simulink model "Gantry1DSimulink_V4"  (R2024b)
settings: Solver=FixedStepAuto  StartTime=0.0  StopTime=inf  FixedStep=0.05  RelTol=1e-3  EnableMultiTasking=on
undefined symbols (not defined in the file): DiscIntNeverNeededParam
libraries: raspberrypiBasiclib x5, raspberrypiNetworklib x5, etargetslib x1, simulink x1
settings Model: ExtModeTrigDuration=2  Creator=ioannisgeorgilas  LastModifiedBy=oskarchu
settings SolverCC: PositivePriorityOrder=on
settings OptimizationCC: EnhancedBackFolding=on  PassReuseOutputArgsAs=Individual arguments  ZeroExternalMemoryAtStartup=off  ZeroInternalMemoryAtStartup=off  MaxStackSize=200000  OptimizeBlockOrder=speed  DifferentSizesBufferReuse=on  OptimizationCustomize=off  EfficientTunableParamExpr=on
settings DebuggingCC: ParameterTunabilityLossMsg=error
settings HardwareCC: ProdBitPerPointer=32  ProdBitPerSizeT=32  ProdBitPerPtrDiffT=32  ProdLargestAtomicInteger=Long  ProdLargestAtomicFloat=Double  ProdWordSize=32  ProdLongLongMode=on  ProdHWDeviceType=ARM Compatible->ARM Cortex-A (32-bit)
settings RTWCC: Description=Embedded Coder  SystemTargetFile=ert.tlc  HardwareBoard=Raspberry Pi  TLCOptions="-aInlineSetEventsForThisBaseRateFcn=TLC_FALSE -aSuppressMultiTaskScheduler=TLC_FALSE  -aRateBasedStepFcn=0"  TemplateMakefile=ert_default_tmf  Toolchain=GNU GCC Embedded Linux  BuildConfiguration=Faster Runs
settings CodeAppCC: ForceParamTrailComments=on  IgnoreCustomStorageClasses=off  OperatorAnnotations=on  SimulinkDataObjDesc=on  SFDataObjDesc=on  InsertBlockDesc=on
settings ERTTargetCC: CodeReplacementLibrary=ARM Cortex-A CMSIS  SupportVariableSizeSignals=on  ExtModeTransport=2  ExtModeStaticAlloc=on  ExtModeMexFile=ext_xcp  ExtModeIntrfLevel=Level2 - Open  InlinedParameterPlacement=Hierarchical

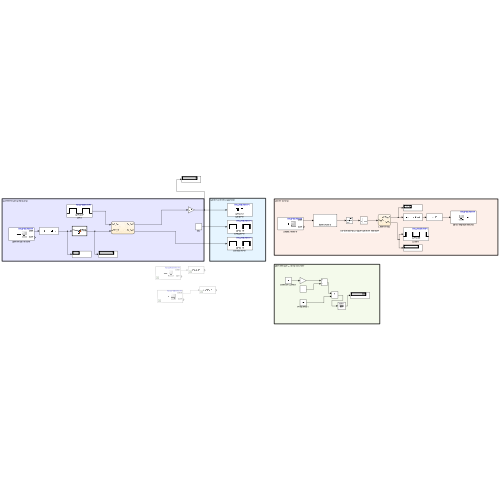
[thumbnail: Simulink's stored preview of the top-level diagram]
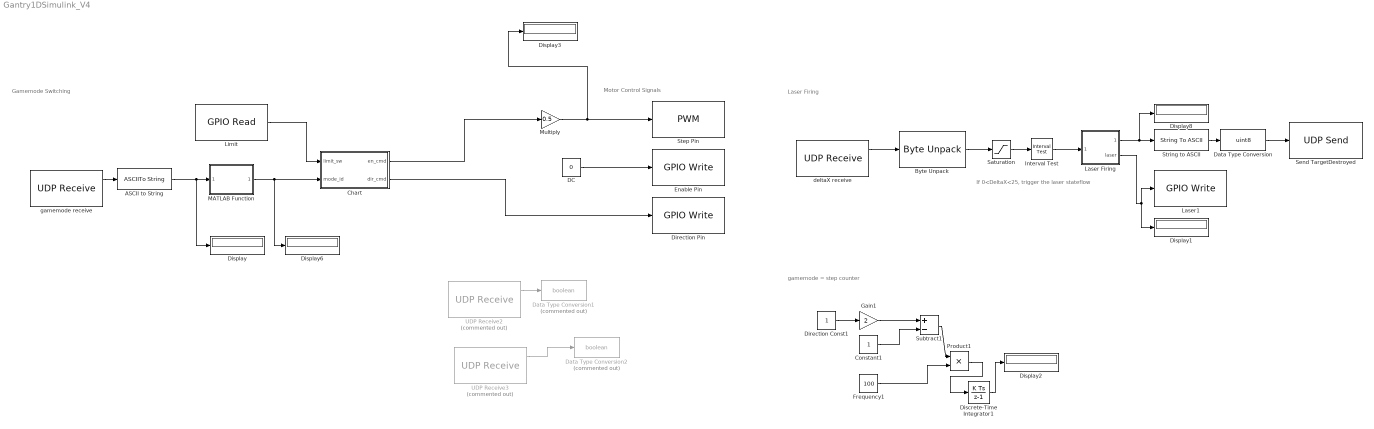
== system Gantry1DSimulink_V4 ==
  note: If 0<DeltaX<25, trigger the laser stateflow
  note: Motor Control Signals
  note: gamemode = step counter
  note: Laser Firing
  note: Gamemode Switching
  ASCII to String : ASCIIToString
  Byte Unpack : etargetslib/Byte Unpack  dimensions={[1]}  datatypes={'int32'}  byteAlign=1
      settings: LibrarySourceBlock=embeddedtargetslib/Host Communication/Byte Unpack
  Chart : Stateflow chart  TreatAsAtomicUnit=on
  Constant1 : Constant
  DC : Constant  Value=0
  Data Type Conversion : DataTypeConversion  OutDataTypeStr=uint8  SaturateOnIntegerOverflow=off  RndMeth=Floor
  Data Type Conversion1 : DataTypeConversion  Commented=on  OutDataTypeStr=boolean  SaturateOnIntegerOverflow=off  RndMeth=Floor
  Data Type Conversion2 : DataTypeConversion  Commented=on  OutDataTypeStr=boolean  SaturateOnIntegerOverflow=off  RndMeth=Floor
  Direction Const1 : Constant
  Direction Pin : raspberrypiBasiclib/GPIO Write  BoardProperty=Pi Zero 2 W  gpio=14  blockPlatform=Raspberry Pi  PinNumber=17  board=[]  direction=[]
  Discrete-Time Integrator1 : DiscreteIntegrator  SampleTime=-1  ICPrevOutput=DiscIntNeverNeededParam  ICPrevScaledInput=DiscIntNeverNeededParam
  Display{,1..3,6,8} (6 alike) : Display
  Enable Pin : raspberrypiBasiclib/GPIO Write  BoardProperty=Pi Zero 2 W  gpio=19  blockPlatform=Raspberry Pi  PinNumber=17  board=[]  direction=[]
  Frequency1 : Constant  Value=100
  Gain1 : Gain  Gain=2
  Interval Test : simulink/Logic and Bit Operations/Interval Test  IntervalClosedRight=on  uplimit=25  IntervalClosedLeft=on  lowlimit=0  OutDataTypeStr=boolean
  Laser Firing : Stateflow chart  TreatAsAtomicUnit=on
  Laser1 : raspberrypiBasiclib/GPIO Write  BoardProperty=Pi Zero 2 W  gpio=22  blockPlatform=Raspberry Pi  PinNumber=17  board=[]  direction=[]
  Limit : raspberrypiBasiclib/GPIO Read  BoardProperty=Pi Zero 2 W  gpio=27  SampleTime=0.05  blockPlatform=Raspberry Pi  PinNumber=4  board=[]  direction=[]  internalResistor=[]
  MATLAB Function : MATLAB Function  TreatAsAtomicUnit=on
  Multiply : Gain  Gain=0.5
  Product1 : Product
  Saturation : Saturate  UpperLimit=500  LowerLimit=-500
  Send TargetDestroyed : raspberrypiNetworklib/UDP Send  remoteURL='172.26.236.65'  remotePort=55004  localURL='0.0.0.0'  localPortSource=Automatically determine  localPort=-1  sampletime=-1  blockPlatform=Raspberry Pi  separateLengthPort=0
      settings: SourceProductName=Network
  Step Pin : raspberrypiBasiclib/PWM  board=Pi Zero W  Pin_=12  Frequency=200  blockPlatform=Raspberry Pi
  String to ASCII : StringToASCII
  Subtract1 : Sum  Inputs=+-
  UDP Receive2 : raspberrypiNetworklib/UDP Receive  Commented=on  localURL='0.0.0.0'  localPort=50001  remoteURL='0.0.0.0'  remotePort=-1  recvBufferSize=8192  signalDatatype=uint8  dims=1  isVarSize=off  showBlockingTime=off  blockingTime=0  sampletime=1  blockPlatform=Raspberry Pi
      settings: SourceProductName=Network
  UDP Receive3 : raspberrypiNetworklib/UDP Receive  Commented=on  localURL='0.0.0.0'  localPort=50002  remoteURL='0.0.0.0'  remotePort=-1  recvBufferSize=8192  signalDatatype=uint8  dims=1  isVarSize=off  showBlockingTime=off  blockingTime=0  sampletime=1  blockPlatform=Raspberry Pi
      settings: SourceProductName=Network
  deltaX receive : raspberrypiNetworklib/UDP Receive  localURL='0.0.0.0'  localPort=55010  remoteURL='0.0.0.0'  remotePort=-1  recvBufferSize=8192  signalDatatype=uint8  dims=4  isVarSize=off  showBlockingTime=off  blockingTime=0  sampletime=0.05  blockPlatform=Raspberry Pi
      settings: SourceProductName=Network
  gamemode receive : raspberrypiNetworklib/UDP Receive  localURL='0.0.0.0'  localPort=50001  remoteURL='0.0.0.0'  remotePort=-1  recvBufferSize=8192  signalDatatype=uint8  dims=14  isVarSize=off  showBlockingTime=off  blockingTime=0  sampletime=0.05  blockPlatform=Raspberry Pi
      settings: SourceProductName=Network
  wires:
  UDP Receive3/1 -> Data Type Conversion2/1
  UDP Receive2/1 -> Data Type Conversion1/1
  Chart/2(dir_cmd) -> Direction Pin/1
  Discrete-Time Integrator1/1 -> Display2/1
  Product1/1 -> Discrete-Time Integrator1/1
  Direction Const1/1 -> Gain1/1
  Frequency1/1 -> Product1/2
  Subtract1/1 -> Product1/1
  Constant1/1 -> Subtract1/2
  Gain1/1 -> Subtract1/1
  ASCII to String/1 -> MATLAB Function/1(command_string), Display/1
  Limit/1 -> Chart/1(limit_sw)
  Multiply/1 -> Display3/1, Step Pin/1
  DC/1 -> Enable Pin/1
  MATLAB Function/1(mode_id) -> Chart/2(mode_id), Display6/1
  gamemode receive/1 -> ASCII to String/1
  deltaX receive/1 -> Byte Unpack/1
  Byte Unpack/1 -> Saturation/1
  Interval Test/1 -> Laser Firing/1(trigger)
  Laser Firing/2(laser) -> Display1/1, Laser1/1
  Saturation/1 -> Interval Test/1
  Data Type Conversion/1 -> Send TargetDestroyed/1
  Laser Firing/1(message) -> Display8/1, String to ASCII/1
  String to ASCII/1 -> Data Type Conversion/1
  Chart/1(en_cmd) -> Multiply/1

== stateflow chart Gantry1DSimulink_V4/Laser Firing ==
  state Idle
    entry: laser = 0;
    entry: message = "Idle";
  state Fire
    entry: laser = 1;
    entry: message = "Firing";
  state Send
    entry: message = "Target Destroyed";
  (default) -> Idle
  Idle -> Fire : [trigger == 1]
  Send -> Idle : [after(1, sec)]
  Fire -> Send : after(5, sec)
  data: message output string; laser output; trigger input

== matlab function Gantry1DSimulink_V4/MATLAB Function ==
  data: command_string input; mode_id output
function mode_id = fcn(command_string)
    % Input: command_string (from 'ASCII to String' block)
    % Output: Integer ID for Stateflow
    
    % Convert the Simulink string to a character array
    cmd_chars = char(command_string);
    
    % Safety Check: If empty, do nothing (Idle)
    if isempty(cmd_chars)
        mode_id = 0;
        return;
    end
    
    % Grab just the first letter
    first_letter = cmd_chars(1);
    
    % Check logic
    if first_letter == 'i'      % i = idle
        mode_id = 0;
        
    elseif first_letter == 'c'  % c = calibrate
        mode_id = 1;
        
    elseif first_letter == 's'  % f = selection
        mode_id = 2;
        
    elseif first_letter == 'a'  % a = attack
        mode_id = 3;
        
    elseif first_letter == 'e'  % e = end
        mode_id = 4;
        
    else
        % Default to Idle if unknown
        mode_id = 0; 
    end
end

== stateflow chart Gantry1DSimulink_V4/Chart ==
  state MoveAway
    entry: en_cmd = 1;
    entry: dir_cmd = 1;
  state MoveHome
    entry: en_cmd = 1;
    entry: dir_cmd = 0;
  state idle
    entry: en_cmd = 0;
    entry: dir_cmd = 0;
  state Attack
    entry: en_cmd = 1;
    entry: dir_cmd = 0;
  state idle1
    entry: en_cmd = 0;
    entry: dir_cmd = 0;
  state Finding
    entry: en_cmd = 1;
    entry: dir_cmd = 1;
  state idle2
    entry: en_cmd = 0;
    entry: dir_cmd = 0;
  idle -> MoveAway : [mode_id == 1]
  MoveAway -> MoveHome : after(2, sec)
  (default) -> idle
  Attack -> idle : [limit_sw == 0]
  MoveHome -> idle1 : [limit_sw == 0]
  idle2 -> Attack : [mode_id == 3]
  idle1 -> Finding : [mode_id == 2]
  Finding -> idle2 : after(10, sec)
  data: limit_sw input; en_cmd output double =1; dir_cmd output =1; mode_id input
